simulink model "sekwencja_moore"  (R2015a)
settings: Solver=ode45  StartTime=0.0  StopTime=10  RelTol=1e-3
undefined symbols (not defined in the file): sigbuilder_block
settings Model: Creator=Student  LastModifiedBy=lenovo

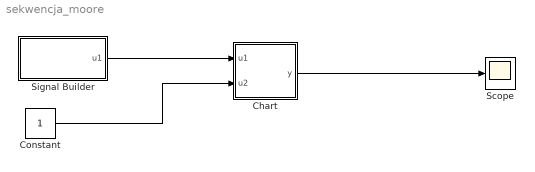
== system sekwencja_moore ==
  Chart : Stateflow chart  TreatAsAtomicUnit=on
  Constant : Constant
  Scope : Scope
      settings: YMin=-0.5  YMax=1.5
  Signal Builder : Subsystem  Tag=STV Subsys  LoadFcn=sigbuilder_block('load',[437.25 153 551.25 360 ]);  StartFcn=sigbuilder_block('start');  StopFcn=sigbuilder_block('stop');  ClipboardFcn=sigbuilder_block('clipboard');  mask(Sigbuilder block){}
      mask help: Simulink:masks:SigbuilderBlock_MD
      mask init:
      | if ~strcmp(get_param(bdroot(gcbh),'SimulationStatus'),'stopped') tuvar = sigbuilder_block('maskInit'); end
      settings: CopyFcn=sigbuilder_block('copy');  DeleteFcn=sigbuilder_block('delete');  ModelCloseFcn=sigbuilder_block('modelClose');  PreSaveFcn=sigbuilder_block('preSave');  PauseFcn=sigbuilder_block('pause');  ContinueFcn=sigbuilder_block('continue');  NameChangeFcn=sigbuilder_block('namechange');  OpenFcn=sigbuilder_block('open',[437.6 199.2 550.4 400 ]);  CloseFcn=sigbuilder_block('close');
      mask Display: plot(0, 0, 100, 100,[2, 2, 32, 32, 2], [68, 8, 8, 68, 68],[32, 2], [38, 38], [32, 19, 2],[53, 60, 44], [32, 17, 17, 2],[16, 16, 31, 31]);txt = getActiveGroup(gcbh);text(2, 100, txt,'verticalAlignment', 'top');
  wires:
  Chart/1(y) -> Scope/1
  Constant/1 -> Chart/2(u2)
  Signal Builder/1(u1) -> Chart/1(u1)

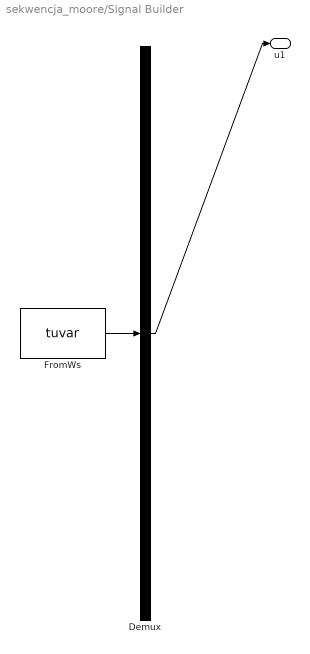
== system sekwencja_moore/Signal Builder ==
  Demux : Demux  Tag=STV Demux  Outputs=1
  FromWs : FromWorkspace  Tag=STV FromWs  VariableName=tuvar  SampleTime=0
      SigBuilderData=|
      | common.afterFinalStr = 'Extrapolate'
      | common.sampleTime = 0
      | dataSet.timeRange = [0 10]
      | dataSet.name = 'Group 1'
      | sbobj.Groups.Name = 'Group 1'
      | sbobj.Groups.Signals.Name = 'u1'
      | sbobj.Groups.Signals.XData = [0 0.5 1 1 1.5 1.5 2 2.5 2.5 3 3.5 4 4.5 5 5 5.5 6 6.5 6.5 7 7 7.5 7.5 8 8 8.5 8.5 9 9 9.5 9.5 10]
      | sbobj.Groups.Signals.YData = [0 0 0 1 1 2 2 2 3 3 3 3 3 3 1 1 1 1 0 0 1 1 2 2 3 3 1 1 1.05 1.05 0 0]
  u1 : Outport  Tag=STV Outport
  wires:
  FromWs/1 -> Demux/1
  Demux/1 -> u1/1

== stateflow chart sekwencja_moore/Chart ==
  settings: stateMachineType=MOORE_MACHINE
  state stan2
    y=0;
  state stan6
    y=1;
  state stan3
    y=0;
  state stan5
    y=0;
  state stan1
    y=0;
  state stan4
    y=0;
  (default) -> stan1
  stan2 -> stan3 [order 2] : [u1==2]
  stan3 -> stan4 [order 2] : [u2==1]
  stan4 -> stan5 [order 1] : [u1==3]
  stan1 -> stan2 [order 1] : [u1==1]
  stan1 -> stan1 [order 2] : [u1~=1]
  stan5 -> stan6 [order 1] : [u1==1]
  stan2 -> stan1 [order 1] : [u1~=2]
  stan6 -> stan1
  stan3 -> stan1 [order 1] : [u2~=1]
  stan5 -> stan1 [order 2] : [u1~=1]
  stan4 -> stan1 [order 2] : [u1~=3]
  data: u1 input; y output; u2 input
